simulink model "SineWaveZeroCondition"  (R2017a)
settings: Solver=VariableStepAuto  StartTime=0.0  StopTime=20  RelTol=1e-3
settings Model: Creator=drone  LastModifiedBy=drone
settings DataIOCC: SaveFinalState=on  SaveFormat=Array  SaveState=on

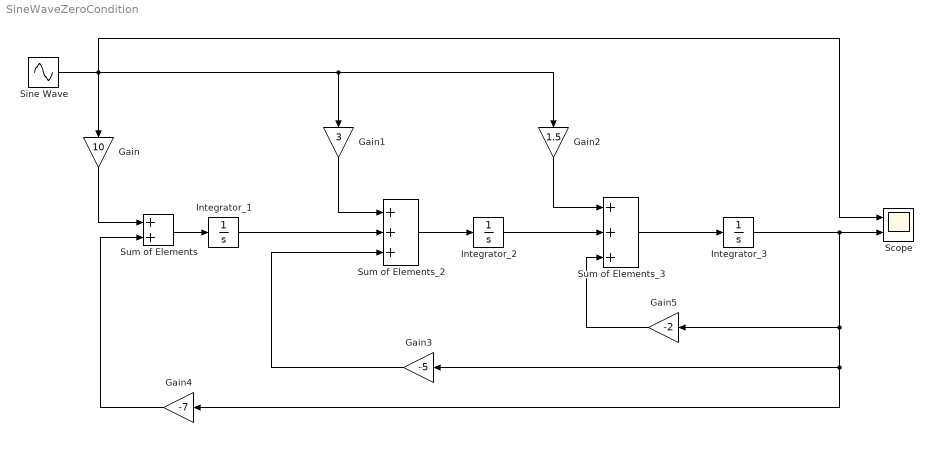
== system SineWaveZeroCondition ==
  Gain : Gain  Gain=10
  Gain1 : Gain  Gain=3
  Gain2 : Gain  Gain=1.5
  Gain3 : Gain  Gain=-5
  Gain4 : Gain  Gain=-7
  Gain5 : Gain  Gain=-2
  Integrator_1 : Integrator
  Integrator_2 : Integrator
  Integrator_3 : Integrator
  Scope : Scope  NumInputPorts=2
  Sine Wave : Sin  Amplitude=2  SampleTime=0
  Sum of Elements : Sum
  Sum of Elements_2 : Sum  Inputs=+++
  Sum of Elements_3 : Sum  Inputs=+++
  wires:
  Sine Wave/1 -> Gain1/1, Gain2/1, Gain/1, Scope/1
  Sum of Elements/1 -> Integrator_1/1
  Integrator_1/1 -> Sum of Elements_2/2
  Gain1/1 -> Sum of Elements_2/1
  Gain2/1 -> Sum of Elements_3/1
  Sum of Elements_3/1 -> Integrator_3/1
  Gain/1 -> Sum of Elements/1
  Gain4/1 -> Sum of Elements/2
  Integrator_3/1 -> Scope/2, Gain4/1, Gain3/1, Gain5/1
  Gain3/1 -> Sum of Elements_2/3
  Gain5/1 -> Sum of Elements_3/3
  Sum of Elements_2/1 -> Integrator_2/1
  Integrator_2/1 -> Sum of Elements_3/2
